simulink model "A1_actuation"  (R2024b)
settings: Solver=ode4  StartTime=0  StopTime=T_final  FixedStep=h  RelTol=1e-3
StopFcn:
  | A1_plot;
values from neighbouring files (symbols this model uses):
  animate = 1    [A1_0_setup.m]
  B_alloc = cfg.B    [A1_0_setup.m]
  beta_c = 0    [A1_0_setup.m]
  h = 0.02    [A1_0_setup.m]    (also in A1_1_build_actuation.m = Simulink.Annotation([m '/note']))
  k_neg = cfg.k_neg    [A1_0_setup.m]
  k_pos = cfg.k_pos    [A1_0_setup.m]
  mp = 25    [A1_0_setup.m]
  n_cmd = [60; -60]    [A1_0_setup.m]
  n_max = cfg.n_max    [A1_0_setup.m]
  n_min = cfg.n_min    [A1_0_setup.m]
  rp = [0.05 0 -0.35]'    [A1_0_setup.m]
  V_c = 0    [A1_0_setup.m]
  x0 = zeros(12,1)    [A1_0_setup.m]    (also in A1_F_sway_without_force.m)
settings Model: Creator=admin  LastModifiedBy=admin
settings DataIOCC: ReturnWorkspaceOutputs=off

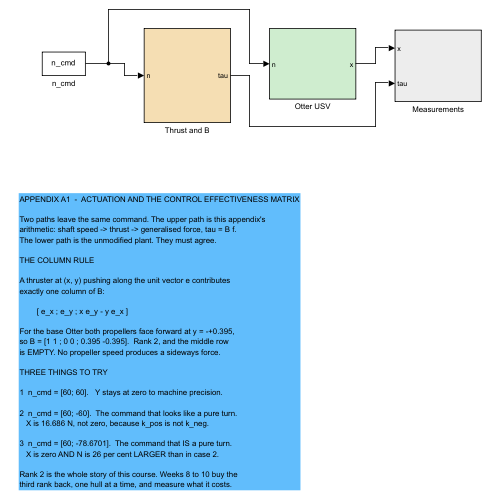
[thumbnail: Simulink's stored preview of the top-level diagram]
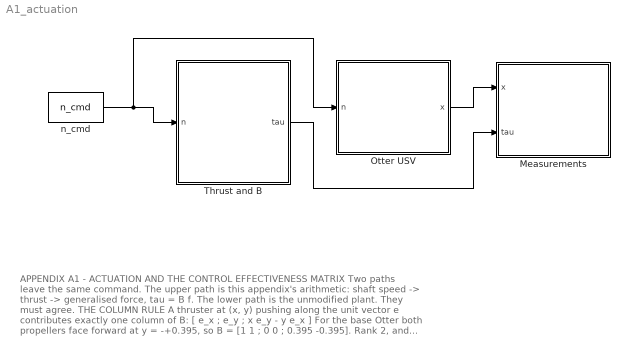
== system A1_actuation ==
  note: APPENDIX A1  -  ACTUATION AND THE CONTROL EFFECTIVENESS MATRIX
      |
      | Two paths leave the same command. The upper path is this appendix's
      | arithmetic: shaft speed -> thrust -> generalised force, tau = B f.
      | The lower path is the unmodified plant. They must agree.
      |
      | THE COLUMN RULE
      |
      | A thruster at (x, y) pushing along the unit vector e contributes
      | exactly one column of B:
      |
      |         [ e_x ; e_y ; x e_y - y e_x ]
      |
      | For the base Otter both propellers face forward at y = -+0.395,
      | so B = [1 1 ; 0 0 ; 0.395 -0.395].  Rank 2, and the middle row
      | is EMPTY. No propeller speed produces a sideways force.
      |
      | THREE THINGS TO TRY
      |
      | 1  n_cmd = [60; 60].   Y stays at zero to machine precision.
      |
      | 2  n_cmd = [60; -60].  The command that looks like a pure turn.
      |    X is 16.686 N, not zero, because k_pos is not k_neg.
      |
      | 3  n_cmd = [60; -78.6701].  The command that IS a pure turn.
      |    X is zero AND N is 26 per cent LARGER than in case 2.
      |
      | Rank 2 is the whole story of this course. Weeks 8 to 10 buy the
      | third rank back, one hull at a time, and measure what it costs.
  Measurements : Subsystem
  Otter USV : Subsystem
  Thrust and B : Subsystem
  n_cmd : Constant  Value=n_cmd
  wires:
  n_cmd/1 -> Thrust and B/1(n), Otter USV/1(n)
  Otter USV/1(x) -> Measurements/1(x)
  Thrust and B/1(tau) -> Measurements/2(tau)

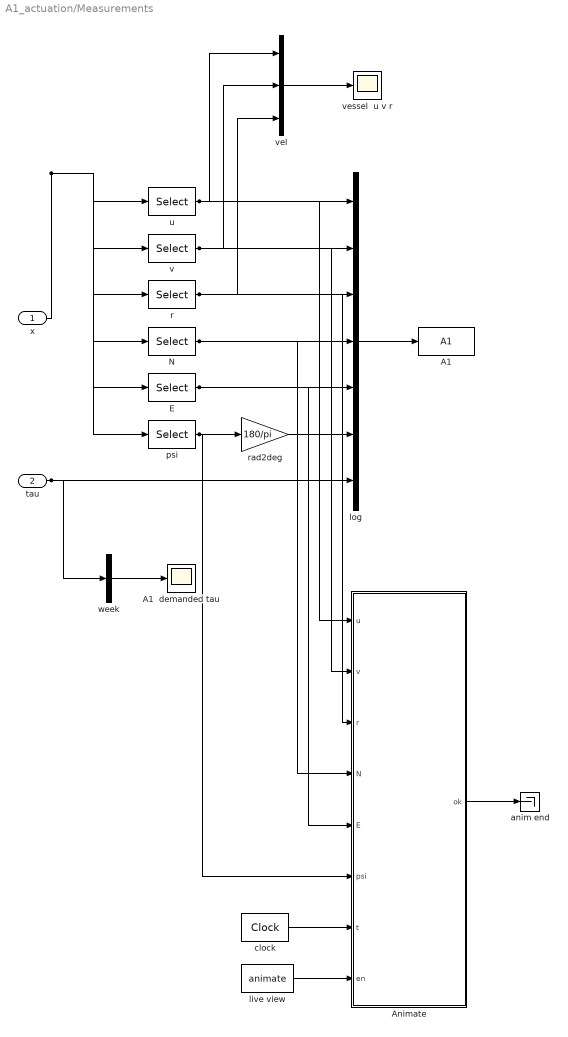
== system A1_actuation/Measurements ==
  x : Inport
  tau : Inport  Port=2
  A1 : ToWorkspace  VariableName=A1  SaveFormat=Structure With Time  SampleTime=-1
  A1  demanded tau : Scope
  Animate : MATLAB Function  TreatAsAtomicUnit=on
  E : Selector  InputPortWidth=12  IndexOptions=Index vector (dialog)  Indices=8  OutputSizes=1
  N : Selector  InputPortWidth=12  IndexOptions=Index vector (dialog)  Indices=7  OutputSizes=1
  anim end : Terminator
  clock : DigitalClock  SampleTime=h
  live view : Constant  Value=animate
  log : Mux  Inputs=7
  psi : Selector  InputPortWidth=12  IndexOptions=Index vector (dialog)  Indices=12  OutputSizes=1
  r : Selector  InputPortWidth=12  IndexOptions=Index vector (dialog)  Indices=6  OutputSizes=1
  rad2deg : Gain  Gain=180/pi
  u : Selector  InputPortWidth=12  IndexOptions=Index vector (dialog)  Indices=1  OutputSizes=1
  v : Selector  InputPortWidth=12  IndexOptions=Index vector (dialog)  Indices=2  OutputSizes=1
  vel : Mux  Inputs=3
  vessel  u v r : Scope
  week : Mux  Inputs=1
  wires:
  x/1 -> u/1, v/1, r/1, N/1, E/1, psi/1
  log/1 -> A1/1
  psi/1 -> rad2deg/1, Animate/6(psi)
  u/1 -> log/1, vel/1, Animate/1(u)
  v/1 -> log/2, vel/2, Animate/2(v)
  r/1 -> log/3, vel/3, Animate/3(r)
  N/1 -> log/4, Animate/4(N)
  E/1 -> log/5, Animate/5(E)
  rad2deg/1 -> log/6
  tau/1 -> log/7, week/1
  vel/1 -> vessel  u v r/1
  week/1 -> A1  demanded tau/1
  clock/1 -> Animate/7(t)
  live view/1 -> Animate/8(en)
  Animate/1(ok) -> anim end/1

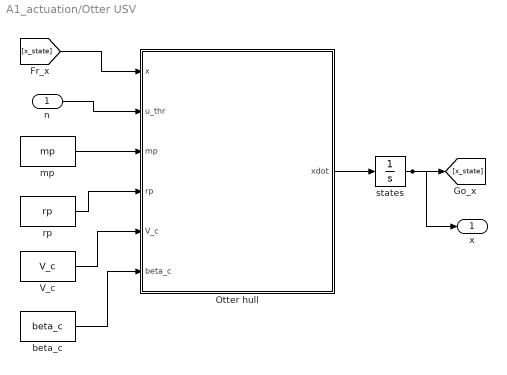
== system A1_actuation/Otter USV ==
  n : Inport
  Otter hull : MATLAB Function  TreatAsAtomicUnit=on
  V_c : Constant  Value=V_c
  beta_c : Constant  Value=beta_c
  mp : Constant  Value=mp
  rp : Constant  Value=rp
  states : Integrator  InitialCondition=x0
  x : Outport
  wires:
  states/1 -> [x_state], x/1
  beta_c/1 -> Otter hull/6(beta_c)
  [x_state] -> Otter hull/1(x)
  n/1 -> Otter hull/2(u_thr)
  mp/1 -> Otter hull/3(mp)
  Otter hull/1(xdot) -> states/1
  rp/1 -> Otter hull/4(rp)
  V_c/1 -> Otter hull/5(V_c)

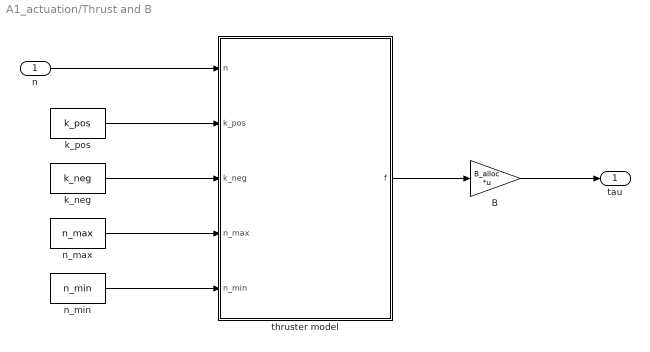
== system A1_actuation/Thrust and B ==
  n : Inport
  B : Gain  Gain=B_alloc  Multiplication=Matrix(K*u)
  k_neg : Constant  Value=k_neg
  k_pos : Constant  Value=k_pos
  n_max : Constant  Value=n_max
  n_min : Constant  Value=n_min
  thruster model : MATLAB Function  TreatAsAtomicUnit=on
  tau : Outport
  wires:
  n/1 -> thruster model/1(n)
  k_pos/1 -> thruster model/2(k_pos)
  k_neg/1 -> thruster model/3(k_neg)
  n_max/1 -> thruster model/4(n_max)
  n_min/1 -> thruster model/5(n_min)
  thruster model/1(f) -> B/1
  B/1 -> tau/1

== matlab function A1_actuation/Otter USV/Otter hull ==
  data: x input; xdot output double size=[12 1]; u_thr input; mp input; rp input; V_c input; beta_c input
function xdot = otter_hull(x, u_thr, mp, rp, V_c, beta_c)
% Fossen's otter.m, called unchanged from Tools/MSS/VESSELS.
%
%   x       12 states, fed back from the integrator
%   u_thr   propeller shaft speeds [rad/s]
%
% otter.m is not written for code generation, so the call is extrinsic and
% xdot has to be pre-sized for Simulink to know the output width.
coder.extrinsic('otter');

xdot = zeros(12,1);
xdot = otter(x, u_thr, mp, rp, V_c, beta_c);
end

== matlab function A1_actuation/Thrust and B/thruster model ==
  data: n input; f output double size=[2 1]; k_pos input; k_neg input; n_max input; n_min input
function f = thruster(n, k_pos, k_neg, n_max, n_min)
%#codegen
% Shaft speed to thrust, one propeller at a time.
%
%   T = k n|n|,  with k_pos going ahead and k_neg going astern.
%
% The saturation is applied to n and NOT to T. A propeller is limited by what
% the motor can turn, not by the force the naval architect would like.
f = zeros(2,1);
for i = 1:2
    ni = min(max(n(i), n_min), n_max);
    if ni >= 0
        f(i) = k_pos * ni * abs(ni);
    else
        f(i) = k_neg * ni * abs(ni);
    end
end
end

== matlab function A1_actuation/Measurements/Animate ==
  data: u input; ok output; v input; r input; N input; E input; psi input; t input; en input
function ok = Animate(u, v, r, N, E, psi, t, en)
%#codegen
% Live view of the vessel while the model runs.
%
% A MATLAB Function block cannot plot, so the drawing function is declared
% extrinsic: Simulink calls plain MATLAB rather than generating code for it.
% Set animate = 0 in the setup script to switch the live view off.
%
% psi arrives in RADIANS and r in rad/s - the units otter.m works in. The
% wrapper converts them for display, in one place, so no two figures in the
% course can disagree about what a degree is.
coder.extrinsic('A1_animate');
ok = 1;
if en > 0.5
    A1_animate(u, v, r, N, E, psi, t);
end
end
